simulink model "PMSM_RobotKinematics"  (R2018b)
settings: Solver=VariableStepAuto  StartTime=0.0  StopTime=0.2  FixedStep=Ts  RelTol=1e-4  EnableMultiTasking=on
PreLoadFcn:
  | run('Arm6Assembly_DataFile.m');
model workspace: external: MAT-File E:\SixRobotArm\Simscape_Simulation\StepFile\Arm6Assembly_DataFile.mat (data not in the file)
values from neighbouring files (symbols this model uses):
  smiData =     [Arm6SimscapeData.mat]
undefined symbols (not defined in the file or in its folder): X, Y, Z
libraries: sm_lib x36, fl_lib x25, nesl_utility x19, simulink_extras x7
(part 4 of 4)

== system PMSM_RobotKinematics/Robot/Joint4/Link3_1_RIGID ==
  ReferenceFrame : sm_lib/Frames and Transforms/Reference Frame
  Solid : sm_lib/Body Elements/Solid  InertiaType=Custom  Mass=smiData.Solid(5).mass  MassUnits=kg  CenterOfMass=smiData.Solid(5).CoM  CenterOfMassUnits=mm  MomentsOfInertia=smiData.Solid(5).MoI  MomentsOfInertiaUnits=kg*mm^2  ProductsOfInertia=smiData.Solid(5).PoI  ProductsOfInertiaUnits=kg*mm^2  BasedOnType=DensityFromFile  Density=1000  DensityUnits=kg/m^3  DoExposeReferenceFrame=on  SerializedFrames=<Frames/>  GraphicType=FromGeometry  MarkerShape=Sphere  MarkerSize=10  GraphicVisPropType=SimpleVisualProperties  GraphicDiffuseColor=smiData.Solid(5).color  GraphicSpecularColor=[0.5 0.5 0.5 1.0]  GraphicAmbientColor=[0.15 0.15 0.15 1.0]  GraphicEmissiveColor=[0.0 0.0 0.0 1.0]  GraphicShininess=75  GraphicOpacity=smiData.Solid(5).opacity  GeometryShape=FromFile  RectangleSize=[1 1]  RectangleSizeUnits=m  BrickDimensions=[1 1 1]  BrickDimensionUnits=m  CylinderRadius=1  CylinderRadiusUnits=m  CylinderLength=1  CylinderLengthUnits=m  SphereRadius=1  SphereRadiusUnits=m  EllipsoidRadii=[1 1 1]  EllipsoidRadiiUnits=m  ExtrusionCrossSection=[1 1; -1 1; -1 -1; 1 -1]  ExtrusionCrossSectionUnits=m  ExtrusionLength=1  ExtrusionLengthUnits=m  PolygonNumSides=3  PolygonOuterRadius=1  PolygonOuterRadiusUnits=m  ExtGeomFileType=STEP  ExtGeomFileName=Link3_默认_sldprt.STEP  ExtGeomFileUnits=m  RevolutionCrossSection=[1 1; 1 -1; 2 -1; 2 1]  RevolutionCrossSectionUnits=m  RevolutionExtent=Full  RevolutionAngle=180  RevolutionAngleUnits=deg
  Transform : sm_lib/Frames and Transforms/Rigid Transform  TranslationMethod=Cartesian  TranslationStandardOffset=0  TranslationLengthUnit=mm  TranslationStandardAxis=+Z  TranslationCartesianOffset=smiData.RigidTransform(6).translation  TranslationROffset=0  TranslationROffsetUnits=m  TranslationZOffset=0  TranslationZOffsetUnits=m  TranslationThetaOffset=0  TranslationThetaOffsetUnits=deg  RotationMethod=ArbitraryAxis  RotationAngleUnits=rad  RotationStandardAxis=+Z  RotationAngle=smiData.RigidTransform(6).angle  RotationArbitraryAxis=smiData.RigidTransform(6).axis  FollAlignAxisA=+X  BaseAlignAxisA=+Y  FollAlignAxisB=+Y  BaseAlignAxisB=+Z  RotationSequenceAxes=FollowerAxes  RotationSequence=XYX  RotationSequenceAngles=[0 0 0]  RotationSequenceAnglesUnits=deg  RotationMatrix=[1 0 0; 0 1 0; 0 0 1]
  Transform1 : sm_lib/Frames and Transforms/Rigid Transform  TranslationMethod=Cartesian  TranslationStandardOffset=0  TranslationLengthUnit=mm  TranslationStandardAxis=+Z  TranslationCartesianOffset=smiData.RigidTransform(7).translation  TranslationROffset=0  TranslationROffsetUnits=m  TranslationZOffset=0  TranslationZOffsetUnits=m  TranslationThetaOffset=0  TranslationThetaOffsetUnits=deg  RotationMethod=ArbitraryAxis  RotationAngleUnits=rad  RotationStandardAxis=+Z  RotationAngle=smiData.RigidTransform(7).angle  RotationArbitraryAxis=smiData.RigidTransform(7).axis  FollAlignAxisA=+X  BaseAlignAxisA=+Y  FollAlignAxisB=+Y  BaseAlignAxisB=+Z  RotationSequenceAxes=FollowerAxes  RotationSequence=XYX  RotationSequenceAngles=[0 0 0]  RotationSequenceAnglesUnits=deg  RotationMatrix=[1 0 0; 0 1 0; 0 0 1]
  F : PMIOPort  Side=Left
  F1 : PMIOPort  Port=2  Side=Right
  connections:
  Solid/RConn1 -- ReferenceFrame/RConn1 -- Transform/LConn1 -- Transform1/LConn1
  Transform/RConn1 -- F/RConn1
  Transform1/RConn1 -- F1/RConn1

== system PMSM_RobotKinematics/Robot/Joint5/Link4_1_RIGID ==
  ReferenceFrame : sm_lib/Frames and Transforms/Reference Frame
  Solid : sm_lib/Body Elements/Solid  InertiaType=Custom  Mass=smiData.Solid(1).mass  MassUnits=kg  CenterOfMass=smiData.Solid(1).CoM  CenterOfMassUnits=mm  MomentsOfInertia=smiData.Solid(1).MoI  MomentsOfInertiaUnits=kg*mm^2  ProductsOfInertia=smiData.Solid(1).PoI  ProductsOfInertiaUnits=kg*mm^2  BasedOnType=DensityFromFile  Density=1000  DensityUnits=kg/m^3  DoExposeReferenceFrame=on  SerializedFrames=<Frames/>  GraphicType=FromGeometry  MarkerShape=Sphere  MarkerSize=10  GraphicVisPropType=SimpleVisualProperties  GraphicDiffuseColor=smiData.Solid(1).color  GraphicSpecularColor=[0.5 0.5 0.5 1.0]  GraphicAmbientColor=[0.15 0.15 0.15 1.0]  GraphicEmissiveColor=[0.0 0.0 0.0 1.0]  GraphicShininess=75  GraphicOpacity=smiData.Solid(1).opacity  GeometryShape=FromFile  RectangleSize=[1 1]  RectangleSizeUnits=m  BrickDimensions=[1 1 1]  BrickDimensionUnits=m  CylinderRadius=1  CylinderRadiusUnits=m  CylinderLength=1  CylinderLengthUnits=m  SphereRadius=1  SphereRadiusUnits=m  EllipsoidRadii=[1 1 1]  EllipsoidRadiiUnits=m  ExtrusionCrossSection=[1 1; -1 1; -1 -1; 1 -1]  ExtrusionCrossSectionUnits=m  ExtrusionLength=1  ExtrusionLengthUnits=m  PolygonNumSides=3  PolygonOuterRadius=1  PolygonOuterRadiusUnits=m  ExtGeomFileType=STEP  ExtGeomFileName=Link4_默认_sldprt.STEP  ExtGeomFileUnits=m  RevolutionCrossSection=[1 1; 1 -1; 2 -1; 2 1]  RevolutionCrossSectionUnits=m  RevolutionExtent=Full  RevolutionAngle=180  RevolutionAngleUnits=deg
  Transform : sm_lib/Frames and Transforms/Rigid Transform  TranslationMethod=Cartesian  TranslationStandardOffset=0  TranslationLengthUnit=mm  TranslationStandardAxis=+Z  TranslationCartesianOffset=smiData.RigidTransform(8).translation  TranslationROffset=0  TranslationROffsetUnits=m  TranslationZOffset=0  TranslationZOffsetUnits=m  TranslationThetaOffset=0  TranslationThetaOffsetUnits=deg  RotationMethod=ArbitraryAxis  RotationAngleUnits=rad  RotationStandardAxis=+Z  RotationAngle=smiData.RigidTransform(8).angle  RotationArbitraryAxis=smiData.RigidTransform(8).axis  FollAlignAxisA=+X  BaseAlignAxisA=+Y  FollAlignAxisB=+Y  BaseAlignAxisB=+Z  RotationSequenceAxes=FollowerAxes  RotationSequence=XYX  RotationSequenceAngles=[0 0 0]  RotationSequenceAnglesUnits=deg  RotationMatrix=[1 0 0; 0 1 0; 0 0 1]
  Transform1 : sm_lib/Frames and Transforms/Rigid Transform  TranslationMethod=Cartesian  TranslationStandardOffset=0  TranslationLengthUnit=mm  TranslationStandardAxis=+Z  TranslationCartesianOffset=smiData.RigidTransform(9).translation  TranslationROffset=0  TranslationROffsetUnits=m  TranslationZOffset=0  TranslationZOffsetUnits=m  TranslationThetaOffset=0  TranslationThetaOffsetUnits=deg  RotationMethod=ArbitraryAxis  RotationAngleUnits=rad  RotationStandardAxis=+Z  RotationAngle=smiData.RigidTransform(9).angle  RotationArbitraryAxis=smiData.RigidTransform(9).axis  FollAlignAxisA=+X  BaseAlignAxisA=+Y  FollAlignAxisB=+Y  BaseAlignAxisB=+Z  RotationSequenceAxes=FollowerAxes  RotationSequence=XYX  RotationSequenceAngles=[0 0 0]  RotationSequenceAnglesUnits=deg  RotationMatrix=[1 0 0; 0 1 0; 0 0 1]
  F : PMIOPort  Side=Left
  F1 : PMIOPort  Port=2  Side=Right
  connections:
  Solid/RConn1 -- ReferenceFrame/RConn1 -- Transform/LConn1 -- Transform1/LConn1
  Transform/RConn1 -- F/RConn1
  Transform1/RConn1 -- F1/RConn1

== system PMSM_RobotKinematics/Robot/Joint6/Link5_2_RIGID ==
  ReferenceFrame : sm_lib/Frames and Transforms/Reference Frame
  Solid : sm_lib/Body Elements/Solid  InertiaType=Custom  Mass=smiData.Solid(2).mass  MassUnits=kg  CenterOfMass=smiData.Solid(2).CoM  CenterOfMassUnits=mm  MomentsOfInertia=smiData.Solid(2).MoI  MomentsOfInertiaUnits=kg*mm^2  ProductsOfInertia=smiData.Solid(2).PoI  ProductsOfInertiaUnits=kg*mm^2  BasedOnType=DensityFromFile  Density=1000  DensityUnits=kg/m^3  DoExposeReferenceFrame=on  SerializedFrames=<Frames/>  GraphicType=FromGeometry  MarkerShape=Sphere  MarkerSize=10  GraphicVisPropType=SimpleVisualProperties  GraphicDiffuseColor=smiData.Solid(2).color  GraphicSpecularColor=[0.5 0.5 0.5 1.0]  GraphicAmbientColor=[0.15 0.15 0.15 1.0]  GraphicEmissiveColor=[0.0 0.0 0.0 1.0]  GraphicShininess=75  GraphicOpacity=smiData.Solid(2).opacity  GeometryShape=FromFile  RectangleSize=[1 1]  RectangleSizeUnits=m  BrickDimensions=[1 1 1]  BrickDimensionUnits=m  CylinderRadius=1  CylinderRadiusUnits=m  CylinderLength=1  CylinderLengthUnits=m  SphereRadius=1  SphereRadiusUnits=m  EllipsoidRadii=[1 1 1]  EllipsoidRadiiUnits=m  ExtrusionCrossSection=[1 1; -1 1; -1 -1; 1 -1]  ExtrusionCrossSectionUnits=m  ExtrusionLength=1  ExtrusionLengthUnits=m  PolygonNumSides=3  PolygonOuterRadius=1  PolygonOuterRadiusUnits=m  ExtGeomFileType=STEP  ExtGeomFileName=Link5_默认_sldprt.STEP  ExtGeomFileUnits=m  RevolutionCrossSection=[1 1; 1 -1; 2 -1; 2 1]  RevolutionCrossSectionUnits=m  RevolutionExtent=Full  RevolutionAngle=180  RevolutionAngleUnits=deg
  Transform : sm_lib/Frames and Transforms/Rigid Transform  TranslationMethod=Cartesian  TranslationStandardOffset=0  TranslationLengthUnit=mm  TranslationStandardAxis=+Z  TranslationCartesianOffset=smiData.RigidTransform(10).translation  TranslationROffset=0  TranslationROffsetUnits=m  TranslationZOffset=0  TranslationZOffsetUnits=m  TranslationThetaOffset=0  TranslationThetaOffsetUnits=deg  RotationMethod=ArbitraryAxis  RotationAngleUnits=rad  RotationStandardAxis=+Z  RotationAngle=smiData.RigidTransform(10).angle  RotationArbitraryAxis=smiData.RigidTransform(10).axis  FollAlignAxisA=+X  BaseAlignAxisA=+Y  FollAlignAxisB=+Y  BaseAlignAxisB=+Z  RotationSequenceAxes=FollowerAxes  RotationSequence=XYX  RotationSequenceAngles=[0 0 0]  RotationSequenceAnglesUnits=deg  RotationMatrix=[1 0 0; 0 1 0; 0 0 1]
  Transform1 : sm_lib/Frames and Transforms/Rigid Transform  TranslationMethod=Cartesian  TranslationStandardOffset=0  TranslationLengthUnit=mm  TranslationStandardAxis=+Z  TranslationCartesianOffset=smiData.RigidTransform(11).translation  TranslationROffset=0  TranslationROffsetUnits=m  TranslationZOffset=0  TranslationZOffsetUnits=m  TranslationThetaOffset=0  TranslationThetaOffsetUnits=deg  RotationMethod=ArbitraryAxis  RotationAngleUnits=rad  RotationStandardAxis=+Z  RotationAngle=smiData.RigidTransform(11).angle  RotationArbitraryAxis=smiData.RigidTransform(11).axis  FollAlignAxisA=+X  BaseAlignAxisA=+Y  FollAlignAxisB=+Y  BaseAlignAxisB=+Z  RotationSequenceAxes=FollowerAxes  RotationSequence=XYX  RotationSequenceAngles=[0 0 0]  RotationSequenceAnglesUnits=deg  RotationMatrix=[1 0 0; 0 1 0; 0 0 1]
  F : PMIOPort  Side=Left
  F1 : PMIOPort  Port=2  Side=Right
  connections:
  Solid/RConn1 -- ReferenceFrame/RConn1 -- Transform/LConn1 -- Transform1/LConn1
  Transform/RConn1 -- F/RConn1
  Transform1/RConn1 -- F1/RConn1

== matlab function PMSM_RobotKinematics/MATLAB Function ==
  data: Pos input; AllSloverTheta output
function AllSloverTheta =InverseSolver_MDH(Pos)
%#codegen
%% coder.extrinsic 声明外部函数。
%% 在仿真期间，代码生成器会为外部函数的调用生成代码，但不会生成函数的内部代码。
coder.extrinsic('disp');
%% 建立机器人DH参数，初始状态为竖直状态
%% L1=Link('d',144,'a',0,'alpha',0,'modified'); 
%% L2=Link('d',0,'a',0,'alpha',pi/2,'offset',-pi/2,'modified');
%% L3=Link('d',0,'a',-264,'alpha',0,'modified');
%% L4=Link('d',106,'a',-236,'alpha',0,'offset',-pi/2,'modified');
%% L5=Link('d',114,'a',0,'alpha',pi/2,'modified');
%% L6=Link('d',67,'a',0,'alpha',-pi/2,'modified');
    AllSloverTheta = zeros(8,6);A=zeros(1,4);
    %%        [alpha,a, d,offset] 
    DH_JXB =[0 0 144 0; 
                    90 0 0 -90;
                    0 -264 0 0; 
                    0 -236 106 -90; 
                    90 0 114 0; 
                    -90 0 67 0];
    p2=DH_JXB(2,4);p4=DH_JXB(4,4);
    a2=DH_JXB(3,2);a3=DH_JXB(4,2);d1=DH_JXB(1,3);d4=DH_JXB(4,3);d5=DH_JXB(5,3);
    X=Pos(1);Y=Pos(2);Z=Pos(3);
    gama=Pos(4)*pi/180;beta=Pos(5)*pi/180;alpha=Pos(6)*pi/180;
    theta7=0;a6=0;afa6=0;d7=DH_JXB(6,3);
    T67=[   cos(theta7),-sin(theta7),0,a6;
                sin(theta7)*cos(afa6),cos(theta7)*cos(afa6),-sin(afa6),-sin(afa6)*d7;
                sin(theta7)*sin(afa6),cos(theta7)*sin(afa6),cos(afa6),cos(afa6)*d7;
                0,0,0,1
             ];
   T_goat=[  cos(beta)*cos(gama),-cos(beta)*sin(gama),sin(beta),X;
                   sin(alpha)*sin(beta)*cos(gama)+cos(alpha)*sin(gama), -sin(alpha)*sin(beta)*sin(gama)+cos(alpha)*cos(gama), -sin(alpha)*cos(beta),Y;
                  -cos(alpha)*sin(beta)*cos(gama)+sin(alpha)*sin(gama), cos(alpha)*sin(beta)*sin(gama)+sin(alpha)*cos(gama),  cos(alpha)*cos(beta),Z;
                  0,0,0,1
              ];
    T06=T_goat/T67;
    
    nx=T06(1,1);ny=T06(2,1);
    ox=T06(1,2);oy=T06(2,2);
    ax=T06(1,3);ay=T06(2,3);az=T06(3,3);
    px=T06(1,4);py=T06(2,4);pz=T06(3,4);
    
    k=0;
    ForJudgment=px^2+py^2-d4^2;
    
    if ForJudgment<-1e-6
        disp('Out of workspace Unable to solve');
    else      
        if ForJudgment>=-1e-6&&ForJudgment<0
            ForJudgment=0;
        end
        theta1_1=atan2(py,px)-atan2(-d4,sqrt(ForJudgment));
        theta1_2=atan2(py,px)-atan2(-d4,-sqrt(ForJudgment));
        
        S5_1=sqrt((-sin(theta1_1)*nx+cos(theta1_1)*ny)^2+(-sin(theta1_1)*ox+cos(theta1_1)*oy)^2);
        theta5_1=atan2(S5_1,sin(theta1_1)*ax-cos(theta1_1)*ay);
        S5_2=-sqrt((-sin(theta1_1)*nx+cos(theta1_1)*ny)^2+(-sin(theta1_1)*ox+cos(theta1_1)*oy)^2);
        theta5_2=atan2(S5_2,sin(theta1_1)*ax-cos(theta1_1)*ay);
        S5_3=sqrt((-sin(theta1_2)*nx+cos(theta1_2)*ny)^2+(-sin(theta1_2)*ox+cos(theta1_2)*oy)^2);
        theta5_3=atan2(S5_3,sin(theta1_2)*ax-cos(theta1_2)*ay);
        S5_4=-sqrt((-sin(theta1_2)*nx+cos(theta1_2)*ny)^2+(-sin(theta1_2)*ox+cos(theta1_2)*oy)^2);
        theta5_4=atan2(S5_4,sin(theta1_2)*ax-cos(theta1_2)*ay);
        
        S234 = [0; 0; 0; 0];C234 = [0; 0; 0; 0];
        B = [0; 0; 0; 0];B1 = [0; 0; 0; 0];B2 = [0; 0; 0; 0];
        C = [0; 0; 0; 0];
        theta2 = [0; 0; 0; 0; 0; 0; 0; 0];
        theta23 = [0; 0; 0; 0; 0; 0; 0; 0];
        theta234 = [0; 0; 0; 0; 0; 0; 0; 0];
        theta3 = [0; 0; 0; 0; 0; 0; 0; 0];
        theta4 = [0; 0; 0; 0; 0; 0; 0; 0];
        
        if abs(S5_1)>1e-6
            theta6_1=atan2((-sin(theta1_1)*ox+cos(theta1_1)*oy)/S5_1,(sin(theta1_1)*nx-cos(theta1_1)*ny)/S5_1);
            S234(1)=-az/S5_1;C234(1)=-(cos(theta1_1)*ax+sin(theta1_1)*ay)/S5_1;theta234(1)=atan2(S234(1),C234(1));
            B1(1)=cos(theta1_1)*px+sin(theta1_1)*py-d5*S234(1);B2(1)=pz-d1+d5*C234(1);A(1)=-2*B2(1)*a2;B(1)=2*B1(1)*a2;C(1)=B1(1)^2+B2(1)^2+a2^2-a3^2;
            if A(1)^2+B(1)^2-C(1)^2>=0
                theta2(1)=atan2(B(1),A(1))-atan2(C(1),sqrt(A(1)^2+B(1)^2-C(1)^2));
                theta2(2)=atan2(B(1),A(1))-atan2(C(1),-sqrt(A(1)^2+B(1)^2-C(1)^2));
                theta23(1)=atan2((B2(1)-a2*sin(theta2(1)))/a3,(B1(1)-a2*cos(theta2(1)))/a3);theta23(2)=atan2((B2(1)-a2*sin(theta2(2)))/a3,(B1(1)-a2*cos(theta2(2)))/a3);
                theta4(1)=theta234(1)-theta23(1);
                theta4(2)=theta234(1)-theta23(2);
                theta3(1)=theta23(1)-theta2(1);
                theta3(2)=theta23(2)-theta2(2);
                AllSloverTheta(k+1,:)=[theta1_1 theta2(1)-p2*pi/180 theta3(1) theta4(1)-p4*pi/180 theta5_1 theta6_1];
                AllSloverTheta(k+2,:)=[theta1_1 theta2(2)-p2*pi/180 theta3(2) theta4(2)-p4*pi/180 theta5_1 theta6_1];
                k=k+2;
            end
        end
        if abs(S5_2)>1e-6
            theta6_2=atan2((-sin(theta1_1)*ox+cos(theta1_1)*oy)/S5_2,(sin(theta1_1)*nx-cos(theta1_1)*ny)/S5_2);
            S234(2)=-az/S5_2;C234(2)=-(cos(theta1_1)*ax+sin(theta1_1)*ay)/S5_2;theta234(2)=atan2(S234(2),C234(2));
            B1(2)=cos(theta1_1)*px+sin(theta1_1)*py-d5*S234(2);B2(2)=pz-d1+d5*C234(2);A(2)=-2*B2(2)*a2;B(2)=2*B1(2)*a2;C(2)=B1(2)^2+B2(2)^2+a2^2-a3^2;
            if A(2)^2+B(2)^2-C(2)^2>=0
                theta2(3)=atan2(B(2),A(2))-atan2(C(2),sqrt(A(2)^2+B(2)^2-C(2)^2));
                theta2(4)=atan2(B(2),A(2))-atan2(C(2),-sqrt(A(2)^2+B(2)^2-C(2)^2));
                theta23(3)=atan2((B2(2)-a2*sin(theta2(3)))/a3,(B1(2)-a2*cos(theta2(3)))/a3);theta23(4)=atan2((B2(2)-a2*sin(theta2(4)))/a3,(B1(2)-a2*cos(theta2(4)))/a3);
                theta4(3)=theta234(2)-theta23(3);
                theta4(4)=theta234(2)-theta23(4);
                theta3(3)=theta23(3)-theta2(3);
                theta3(4)=theta23(4)-theta2(4);
                AllSloverTheta(k+1,:)=[theta1_1 theta2(3)-p2*pi/180 theta3(3) theta4(3)-p4*pi/180 theta5_2 theta6_2];
                AllSloverTheta(k+2,:)=[theta1_1 theta2(4)-p2*pi/180 theta3(4) theta4(4)-p4*pi/180 theta5_2 theta6_2];
                k=k+2;
            end
        end
        if abs(S5_3)>1e-6
            theta6_3=atan2((-sin(theta1_2)*ox+cos(theta1_2)*oy)/S5_3,(sin(theta1_2)*nx-cos(theta1_2)*ny)/S5_3);
            S234(3)=-az/S5_3;C234(3)=-(cos(theta1_2)*ax+sin(theta1_2)*ay)/S5_3;theta234(3)=atan2(S234(3),C234(3));
            B1(3)=cos(theta1_2)*px+sin(theta1_2)*py-d5*S234(3);B2(3)=pz-d1+d5*C234(3);A(3)=-2*B2(3)*a2;B(3)=2*B1(3)*a2;C(3)=B1(3)^2+B2(3)^2+a2^2-a3^2;
            if A(3)^2+B(3)^2-C(3)^2>=0
                theta2(5)=atan2(B(3),A(3))-atan2(C(3),sqrt(A(3)^2+B(3)^2-C(3)^2));
                theta2(6)=atan2(B(3),A(3))-atan2(C(3),-sqrt(A(3)^2+B(3)^2-C(3)^2));
                theta23(5)=atan2((B2(3)-a2*sin(theta2(5)))/a3,(B1(3)-a2*cos(theta2(5)))/a3);theta23(6)=atan2((B2(3)-a2*sin(theta2(6)))/a3,(B1(3)-a2*cos(theta2(6)))/a3);
                theta4(5)=theta234(3)-theta23(5);
                theta4(6)=theta234(3)-theta23(6);
                theta3(5)=theta23(5)-theta2(5);
                theta3(6)=theta23(6)-theta2(6);
                AllSloverTheta(k+1,:)=[theta1_2 theta2(5)-p2*pi/180 theta3(5) theta4(5)-p4*pi/180 theta5_3 theta6_3];
                AllSloverTheta(k+2,:)=[theta1_2 theta2(6)-p2*pi/180 theta3(6) theta4(6)-p4*pi/180 theta5_3 theta6_3];
                k=k+2;
            end
        end
        if abs(S5_4)>1e-6
            theta6_4=atan2((-sin(theta1_2)*ox+cos(theta1_2)*oy)/S5_4,(sin(theta1_2)*nx-cos(theta1_2)*ny)/S5_4);
            S234(4)=-az/S5_4;C234(4)=-(cos(theta1_2)*ax+sin(theta1_2)*ay)/S5_4;theta234(4)=atan2(S234(4),C234(4));
            B1(4)=cos(theta1_2)*px+sin(theta1_2)*py-d5*S234(4);B2(4)=pz-d1+d5*C234(4);A(4)=-2*B2(4)*a2;B(4)=2*B1(4)*a2;C(4)=B1(4)^2+B2(4)^2+a2^2-a3^2;
            if A(4)^2+B(4)^2-C(4)^2>=0
                theta2(7)=atan2(B(4),A(4))-atan2(C(4),sqrt(A(4)^2+B(4)^2-C(4)^2));
                theta2(8)=atan2(B(4),A(4))-atan2(C(4),-sqrt(A(4)^2+B(4)^2-C(4)^2));
                theta23(7)=atan2((B2(4)-a2*sin(theta2(7)))/a3,(B1(4)-a2*cos(theta2(7)))/a3);theta23(8)=atan2((B2(4)-a2*sin(theta2(8)))/a3,(B1(4)-a2*cos(theta2(8)))/a3);
                theta4(7)=theta234(4)-theta23(7);
                theta4(8)=theta234(4)-theta23(8);
                theta3(7)=theta23(7)-theta2(7);
                theta3(8)=theta23(8)-theta2(8);
                AllSloverTheta(k+1,:)=[theta1_2 theta2(7)-p2*pi/180 theta3(7) theta4(7)-p4*pi/180 theta5_4 theta6_4];
                AllSloverTheta(k+2,:)=[theta1_2 theta2(8)-p2*pi/180 theta3(8) theta4(8)-p4*pi/180 theta5_4 theta6_4];
                k=k+2;
            end
        end
        
        if k>0
            AllSloverTheta=AllSloverTheta*180/pi;%将弧度转化成角度
            for i=1:k
                for j=1:6
                    if AllSloverTheta(i,j)<=-180
                        AllSloverTheta(i,j)=AllSloverTheta(i,j)+360;%将角度限定在-180—+180
                    elseif AllSloverTheta(i,j)>180
                        AllSloverTheta(i,j)=AllSloverTheta(i,j)-360;%将角度限定在-180—+180
                    end
                end
            end
        else 
                disp('Singular position Unable to solve');
        end
    end
end

== matlab function PMSM_RobotKinematics/MATLAB Function2 ==
  data: Theta input; THETA output
function THETA = round(Theta)
    THETA=[0 0 0 0 0 0; 0 0 0 0 0 0; 0 0 0 0 0 0; 0 0 0 0 0 0; 0 0 0 0 0 0; 0 0 0 0 0 0; 0 0 0 0 0 0; 0 0 0 0 0 0];
    for i=1:8
        for  j=1:6
                if (-1e-6<Theta(i,j)&&Theta(i,j)<0)||(Theta(i,j)>0&&Theta(i,j)<1e-6)
                    Theta(i,j)=0;
                end
                THETA(i,j)=Theta(i,j);
        end
    end
end
